simulink library "giaeb"  (Simulink 8.1)
settings: Solver=ode45  StartTime=0.0  StopTime=10.0  RelTol=1e-3
undefined symbols (not defined in the file or in its folder): FALSE, KIFO_LongAccelNoTargets_mps2, KIFO_RelSpeedNoTargets_kph, KIFO_TargetIdNoTargets_num, KIFO_XPositionNoTargets_m, TRUE, ZERO_INT
libraries: hcu_lib x1
settings Model: Creator=AT015555  LastModifiedBy=AT015555

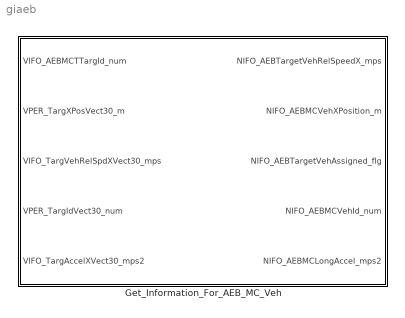
== system giaeb ==
  Get_Information_For_AEB_MC_Veh : Subsystem

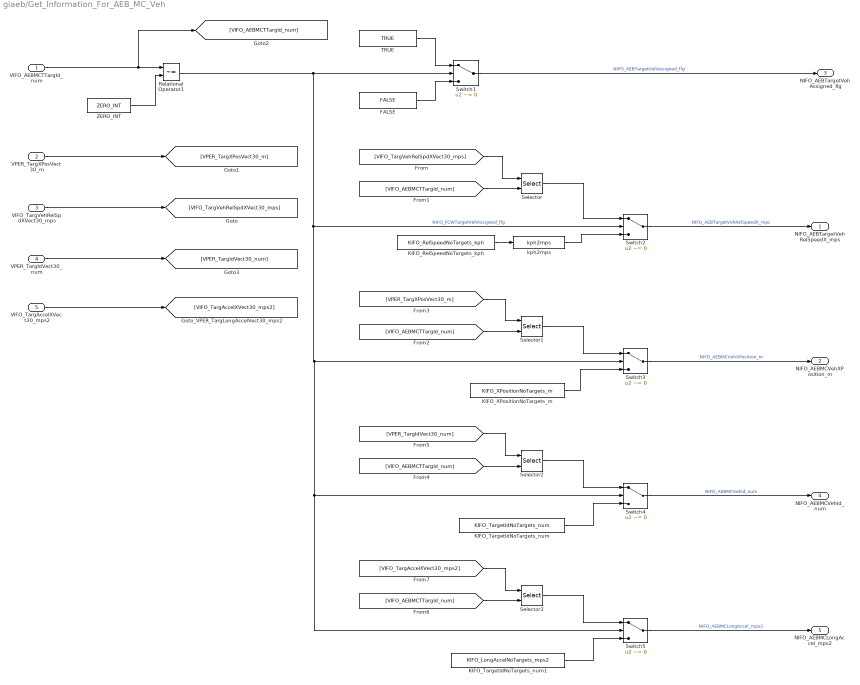
== system giaeb/Get_Information_For_AEB_MC_Veh ==
  VIFO_AEBMCTTargId_num : Inport
  VPER_TargXPosVect30_m : Inport  Port=2
  VIFO_TargVehRelSpdXVect30_mps : Inport  Port=3
  VPER_TargIdVect30_num : Inport  Port=4
  VIFO_TargAccelXVect30_mps2 : Inport  Port=5
  FALSE : Constant  Value=FALSE
  KIFO_RelSpeedNoTargets_kph : Constant  Value=KIFO_RelSpeedNoTargets_kph
  KIFO_TargetIdNoTargets_num : Constant  Value=KIFO_TargetIdNoTargets_num
  KIFO_TargetIdNoTargets_num1 : Constant  Value=KIFO_LongAccelNoTargets_mps2
  KIFO_XPositionNoTargets_m : Constant  Value=KIFO_XPositionNoTargets_m
  Relational Operator1 : RelationalOperator  Operator=~=  OutDataTypeStr=boolean
  Selector{,1..3} (4 alike) : Selector  InputPortWidth=30  IndexOptions=Index vector (port)  Indices=[1 3]  OutputSizes=1
  Switch{1..5} (5 alike) : Switch  Criteria=u2 ~= 0
  TRUE : Constant  Value=TRUE
  ZERO_INT : Constant  Value=ZERO_INT
  kph2mps : hcu_lib/kph2mps
  NIFO_AEBTargetVehRelSpeedX_mps : Outport
  NIFO_AEBMCVehXPosition_m : Outport  Port=2
  NIFO_AEBTargetVehAssigned_flg : Outport  Port=3
  NIFO_AEBMCVehId_num : Outport  Port=4
  NIFO_AEBMCLongAccel_mps2 : Outport  Port=5
  wires:
  Switch3/1 -> NIFO_AEBMCVehXPosition_m/1  "NIFO_AEBMCVehXPosition_m"
  Selector/1 -> Switch2/1
  [VPER_TargXPosVect30_m] -> Selector1/1
  [VIFO_TargVehRelSpdXVect30_mps] -> Selector/1
  FALSE/1 -> Switch1/3
  Switch1/1 -> NIFO_AEBTargetVehAssigned_flg/1  "NIFO_AEBTargetVehAssigned_flg"
  TRUE/1 -> Switch1/1
  ZERO_INT/1 -> Relational Operator1/2
  KIFO_XPositionNoTargets_m/1 -> Switch3/3
  Selector1/1 -> Switch3/1
  VPER_TargXPosVect30_m/1 -> [VPER_TargXPosVect30_m]
  Switch2/1 -> NIFO_AEBTargetVehRelSpeedX_mps/1  "NIFO_AEBTargetVehRelSpeedX_mps"
  [VIFO_AEBMCTTargId_num] -> Selector1/2
  [VIFO_AEBMCTTargId_num] -> Selector/2
  VIFO_TargVehRelSpdXVect30_mps/1 -> [VIFO_TargVehRelSpdXVect30_mps]
  VIFO_AEBMCTTargId_num/1 -> [VIFO_AEBMCTTargId_num], Relational Operator1/1
  KIFO_RelSpeedNoTargets_kph/1 -> kph2mps/1
  VPER_TargIdVect30_num/1 -> [VPER_TargIdVect30_num]
  Switch4/1 -> NIFO_AEBMCVehId_num/1  "NIFO_AEBMCVehId_num"
  [VPER_TargIdVect30_num] -> Selector2/1
  KIFO_TargetIdNoTargets_num/1 -> Switch4/3
  Selector2/1 -> Switch4/1
  [VIFO_AEBMCTTargId_num] -> Selector2/2
  kph2mps/1 -> Switch2/3
  VIFO_TargAccelXVect30_mps2/1 -> [VIFO_TargAccelXVect30_mps2]
  Switch5/1 -> NIFO_AEBMCLongAccel_mps2/1  "NIFO_AEBMCLongAccel_mps2"
  [VIFO_TargAccelXVect30_mps2] -> Selector3/1
  KIFO_TargetIdNoTargets_num1/1 -> Switch5/3
  Selector3/1 -> Switch5/1
  [VIFO_AEBMCTTargId_num] -> Selector3/2
  Relational Operator1/1 -> Switch5/2, Switch4/2, Switch3/2, Switch2/2, Switch1/2  "NIFO_FCWTargetVehAssigned_flg"
